simulink model "lab3"  (R2019a)
settings: Solver=VariableStepAuto  StartTime=0.0  StopTime=200  RelTol=1e-3
settings Model: Creator=sumli  LastModifiedBy=sumli

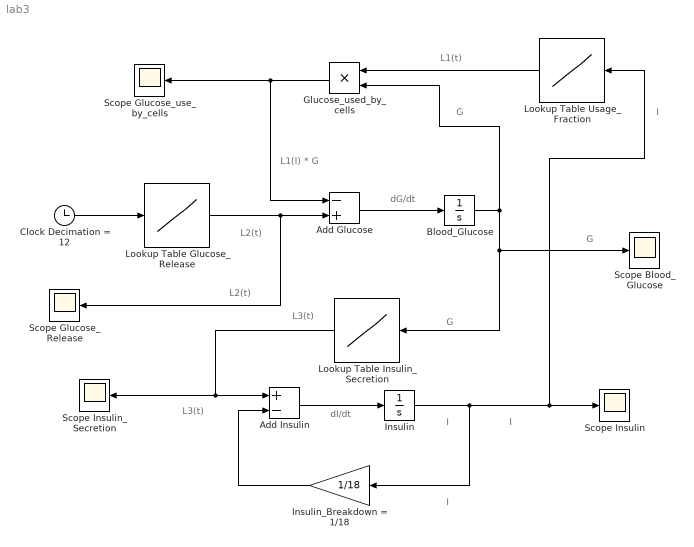
== system lab3 ==
  note: dG/dt
  note: dI/dt
  note: L3(t)
  note: L1(I) * G
  note: L2(t)
  note: I
  note: G
  note: L1(t)
  note: G
  note: L2(t)
  note: G
  note: I
  note: I
  note: I
  note: L3(t)
  Add Glucose : Sum  Inputs=-+
  Add Insulin : Sum  Inputs=+-
  Blood_Glucose : Integrator  InitialCondition=6000
  Clock Decimation = 12 : Clock
  Glucose_used_by_cells : Product
  Insulin : Integrator  InitialCondition=9000
  Insulin_Breakdown = 1/18 : Gain  Gain=1/18
  Lookup Table Glucose_Release : Lookup_n-D  NumberOfTableDimensions=1  BreakpointsForDimension1=[0,12,24,36,48,60,72,84,96,108,120]  Table=[198,198,198,198,198,198,198,198,198,198,198]  InternalRulePriority=Speed  RndMeth=Simplest  InputSameDT=on
  Lookup Table Insulin_Secretion : Lookup_n-D  NumberOfTableDimensions=1  BreakpointsForDimension1=[1000,2000,3000,4000,5000,6000,7000,8000,9000,10000,11000]  Table=[0,15,85,190,350,500,665,825,930,975,995]  InternalRulePriority=Speed  RndMeth=Simplest  InputSameDT=on
  Lookup Table Usage_Fraction : Lookup_n-D  NumberOfTableDimensions=1  BreakpointsForDimension1=[0.00,1800,3600,5400,7200,9000,10800,12600,14400,16200,18000]  Table=[0.0075, 0.0105,0.0145,0.019,0.0255,0.033,0.0405,0.049,0.0545,0.0575,0.059]  InternalRulePriority=Speed  RndMeth=Simplest  InputSameDT=on
  Scope Glucose_use_by_cells : Scope
  Scope Blood_Glucose : Scope
  Scope Glucose_Release : Scope
  Scope Insulin : Scope
  Scope Insulin_Secretion : Scope
  wires:
  Clock Decimation = 12/1 -> Lookup Table Glucose_Release/1
  Lookup Table Glucose_Release/1 -> Scope Glucose_Release/1, Add Glucose/2
  Glucose_used_by_cells/1 -> Add Glucose/1, Scope Glucose_use_by_cells/1
  Add Glucose/1 -> Blood_Glucose/1
  Blood_Glucose/1 -> Lookup Table Insulin_Secretion/1, Scope Blood_Glucose/1, Glucose_used_by_cells/2
  Lookup Table Usage_Fraction/1 -> Glucose_used_by_cells/1
  Insulin/1 -> Insulin_Breakdown = 1/18/1, Lookup Table Usage_Fraction/1, Scope Insulin/1
  Add Insulin/1 -> Insulin/1
  Insulin_Breakdown = 1/18/1 -> Add Insulin/2
  Lookup Table Insulin_Secretion/1 -> Scope Insulin_Secretion/1, Add Insulin/1
